simulink model "usim_model"  (R2023a)
settings: Solver=ode23t  StartTime=0  StopTime=10  RelTol=1e-3  EnableMultiTasking=on
PreLoadFcn:
  | uval = [];
model workspace (MAT data in the model file):
  input_unc = ultidyn
  input_unc.SampleStateDimension = 1
  input_unc.Bound_ = 1
  input_unc.Name_ = 'input_unc'
  input_unc.IOSize_ = [1 1]
  input_unc.Ts_ = 0
  sensor_gain = ureal
  sensor_gain.Mode_ = 'Range'
  sensor_gain.PlusMinus_ = [-0.9 1]
  sensor_gain.NominalValue_ = 1
  sensor_gain.Name_ = 'sensor_gain'
  sensor_gain.IOSize_ = [1 1]
  unc_pole = ureal
  unc_pole.Mode_ = 'Range'
  unc_pole.PlusMinus_ = [-5 1]
  unc_pole.NominalValue_ = -5
  unc_pole.Name_ = 'unc_pole'
  unc_pole.IOSize_ = [1 1]
  wt = ss
  wt.IOSize_ = [1 1]
  wt.Data_ = ltipack.ssdata
  wt.Data_.a = -307.636148721
  wt.Data_.b = 32
  wt.Data_.c = -21.630666707
  wt.Data_.d = 2.5
  wt.Data_.Delay.Input = 0
  wt.Data_.Delay.Output = 0
  wt.Data_.Delay.Internal = []
  wt.Data_.Ts = 0
values from neighbouring files (symbols this model uses):
  input_unc = ultidyn('input_unc',[1 1])    [usim1.m]
  unc_pole = ureal('unc_pole',-5,'Range',[-10 -4])    [usim1.m]
  wt = makeweight(0.25,130,2.5)    [usim1.m]
libraries: RCTblocks x4, simulink x1, cstblocks x1
settings Model: Creator=The MathWorks, Inc.  LastModifiedBy=The MathWorks, Inc.
settings SolverCC: AlgebraicLoopSolver=TrustRegion  MaxZcPerStep=1
settings DataIOCC: LimitDataPoints=on  SaveFormat=Array  ReturnWorkspaceOutputs=off
settings OptimizationCC: DefaultParameterBehavior=Inlined  BufferReuse=off  ExpressionDepthLimit=2147483647  InitFltsAndDblsToZero=on  LifeSpan=inf
settings DebuggingCC: SaveWithParameterizedLinksMsg=none  UnderspecifiedInitializationDetection=Classic  MergeDetectMultiDrivingBlocksExec=none  SignalResolutionControl=TryResolveAllWithWarning  MultiTaskDSMMsg=warning  MultiTaskCondExecSysMsg=none  FcnCallInpInsideContextMsg=warning  UnconnectedInputMsg=warning  UnconnectedOutputMsg=warning  UnconnectedLineMsg=warning  AllowSymbolicDim=off  StateNameClashWarn=warning  SFUnexpectedBacktrackingDiag=warning  SFNoUnconditionalDefaultTransitionDiag=warning  SFExecutionAtInitializationDiag=none  ArithmeticOperatorsInVariantConditions=warning
settings HardwareCC: ProdBitPerPointer=32  ProdBitPerSizeT=32  ProdBitPerPtrDiffT=32  ProdLargestAtomicFloat=None  ProdIntDivRoundTo=Undefined  ProdEndianess=Unspecified  ProdWordSize=32  ProdHWDeviceType=32-bit Generic
settings ModelReferenceCC: EnableRefExpFcnMdlSchedulingChecks=on  PropagateSignalLabelsOutOfModel=off
settings SFSimCC: SimUseLocalCustomCode=off  CustomCodeUndefinedFunction=UseInterfaceOnly
settings RTWCC: RTWUseLocalCustomCode=off
settings CodeAppCC: StateflowObjectComments=on
settings GRTTargetCC: TargetFcnLib=ansi_tfl_tmw.mat  TargetLangStandard=C89/C90 (ANSI)  CombineOutputUpdateFcns=off  GRTInterface=on
settings ConfigComp: CovMetricSettings=dw  CovSaveCumulativeToWorkspaceVar=on  CovSaveSingleToWorkspaceVar=on  CovExternalEMLEnable=off  CovSFcnEnable=off

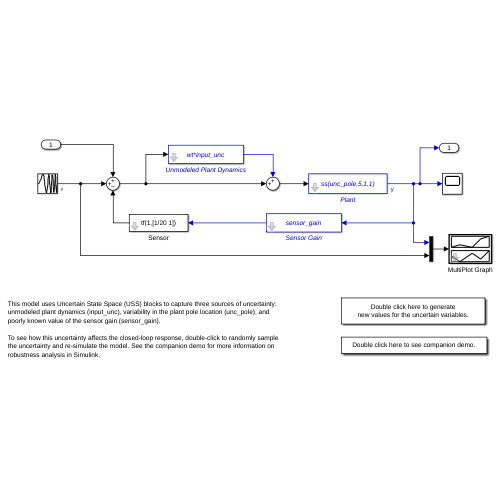
[thumbnail: Simulink's stored preview of the top-level diagram]
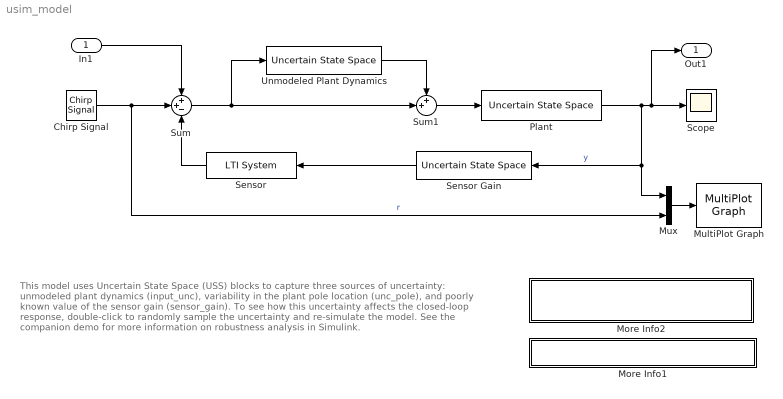
== system usim_model ==
  note: This model uses Uncertain State Space (USS) blocks to capture three sources of uncertainty:
      | unmodeled plant dynamics (input_unc), variability in the plant pole location (unc_pole), and
      | poorly known value of the sensor gain (sensor_gain).
      |
      | To see how this uncertainty affects the closed-loop response, double-click to randomly sample
      | the uncertainty and re-simulate the model. See the companion demo for more information on
      | robustness analysis in Simulink.
  In1 : Inport
  Chirp Signal : simulink/Sources/Chirp Signal  f1=0.1  T=10  f2=1
  More Info1 : Subsystem
      settings: OpenFcn=web(fullfile(matlabroot,'toolbox','robust','rctdemos','html','usim_demo.html'))
      mask Display: fprintf('Double click here to see companion demo.')
  More Info2 : Subsystem
      settings: OpenFcn=uval = usample(ufind(gcs));
      mask Display: disp(sprintf('Double click here to generate\nnew values for the uncertain variables.'))
  MultiPlot Graph : RCTblocks/MultiPlot Graph  Tag=MultiPlot  tmin=0  tmax=10  ymin=[-2 -1.5]  ymax=[2 1.5]  vnamesave=multisimout
  Mux : Mux  Inputs=2
  Plant : RCTblocks/Uncertain State Space  Tag=USS  USystem=ss(unc_pole,5,1,1)  UValue=uval  X0=0  uX0=[0]
  Scope : Scope
  Sensor : cstblocks/LTI System  sys=tf(1,[1/20 1])  IC=[]
  Sensor Gain : RCTblocks/Uncertain State Space  Tag=USS  USystem=sensor_gain  UValue=uval  X0=0  uX0=[0]
  Sum : Sum  Inputs=++-
  Sum1 : Sum  Inputs=++|
  Unmodeled Plant Dynamics : RCTblocks/Uncertain State Space  Tag=USS  USystem=wt*input_unc  UValue=uval  X0=0  uX0=0
  Out1 : Outport  VectorParamsAs1DForOutWhenUnconnected=off
  wires:
  Sensor/1 -> Sum/3
  Chirp Signal/1 -> Sum/2, Mux/2  "r"
  Plant/1 -> Mux/1, Sensor Gain/1, Scope/1, Out1/1  "y"
  Sum1/1 -> Plant/1
  Mux/1 -> MultiPlot Graph/1
  Sensor Gain/1 -> Sensor/1
  Unmodeled Plant Dynamics/1 -> Sum1/1
  Sum/1 -> Sum1/2, Unmodeled Plant Dynamics/1
  In1/1 -> Sum/1

== system usim_model/More Info1 ==

== system usim_model/More Info2 ==
